simulink model "get_pluse_data"  (R2022a)
settings: Solver=FixedStepAuto  StartTime=0.0  StopTime=0.03  FixedStep=0.001  RelTol=1e-3
settings Model: Creator=12496  LastModifiedBy=12496

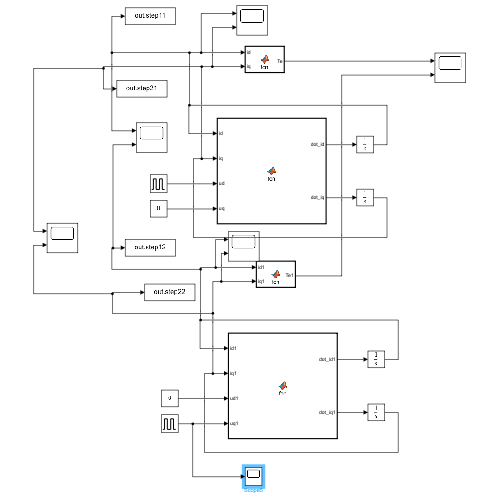
[thumbnail: Simulink's stored preview of the top-level diagram]
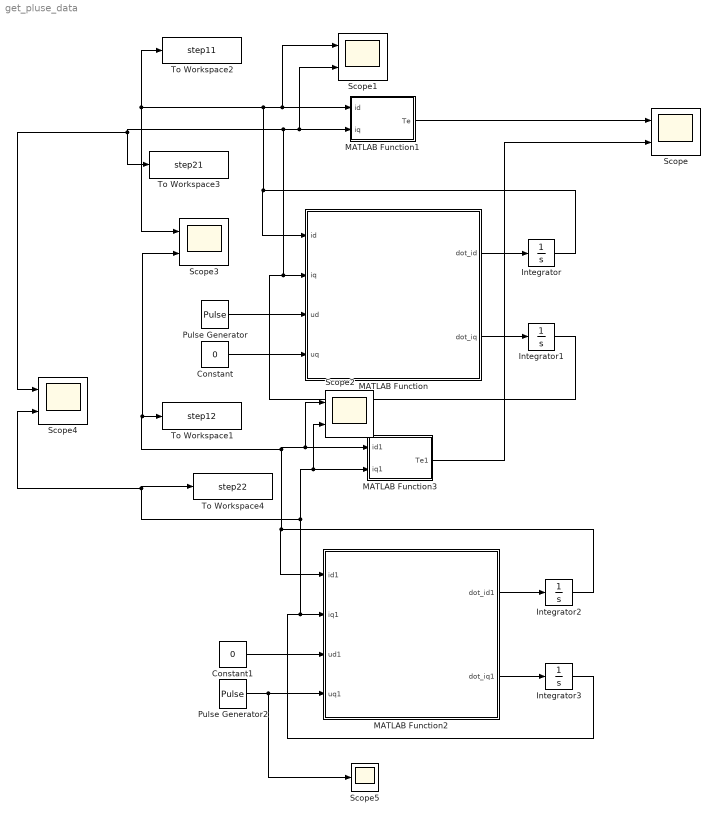
== system get_pluse_data ==
  Constant : Constant  Value=0
  Constant1 : Constant  Value=0
  Integrator{,1..3} (4 alike) : Integrator
  MATLAB Function : MATLAB Function  TreatAsAtomicUnit=on
  MATLAB Function1 : MATLAB Function  TreatAsAtomicUnit=on
  MATLAB Function2 : MATLAB Function  TreatAsAtomicUnit=on
  MATLAB Function3 : MATLAB Function  TreatAsAtomicUnit=on
  Pulse Generator : DiscretePulseGenerator  PulseType=Time based  Period=1  PulseWidth=0.1  PhaseDelay=0.005
  Pulse Generator2 : DiscretePulseGenerator  PulseType=Time based  Period=1  PulseWidth=0.1  PhaseDelay=0.005
  Scope{,1..4} (5 alike) : Scope  NumInputPorts=2
  Scope5 : Scope
  To Workspace1 : ToWorkspace  VariableName=step12  SampleTime=-1
  To Workspace2 : ToWorkspace  VariableName=step11  SampleTime=-1
  To Workspace3 : ToWorkspace  VariableName=step21  SampleTime=-1
  To Workspace4 : ToWorkspace  VariableName=step22  SampleTime=-1
  wires:
  MATLAB Function/1(dot_id) -> Integrator/1
  MATLAB Function/2(dot_iq) -> Integrator1/1
  Pulse Generator/1 -> MATLAB Function/3(ud)
  Constant/1 -> MATLAB Function/4(uq)
  Integrator/1 -> Scope3/1, To Workspace2/1, Scope1/1, MATLAB Function1/1(id), MATLAB Function/1(id)
  Integrator1/1 -> Scope4/1, To Workspace3/1, Scope1/2, MATLAB Function1/2(iq), MATLAB Function/2(iq)
  MATLAB Function1/1(Te) -> Scope/1
  MATLAB Function3/1(Te1) -> Scope/2
  MATLAB Function2/1(dot_id1) -> Integrator2/1
  Integrator2/1 -> MATLAB Function2/1(id1), Scope3/2, To Workspace1/1, Scope2/1, MATLAB Function3/1(id1)
  Integrator3/1 -> Scope4/2, To Workspace4/1, Scope2/2, MATLAB Function3/2(iq1), MATLAB Function2/2(iq1)
  MATLAB Function2/2(dot_iq1) -> Integrator3/1
  Constant1/1 -> MATLAB Function2/3(ud1)
  Pulse Generator2/1 -> Scope5/1, MATLAB Function2/4(uq1)

== matlab function get_pluse_data/MATLAB Function1 ==
  data: id input; Te output; iq input
function Te = fcn(id,iq)
Pn=4; %电机极对数
Fai=0.175; %转子磁链

C = [0 3*Pn*Fai/2];
Te=C*[id;iq];

== matlab function get_pluse_data/MATLAB Function ==
  data: id input; dot_id output; iq input; ud input; uq input; dot_iq output
function [dot_id,dot_iq] = fcn(id,iq,ud,uq)
Ld=0.0085;
Lq=0.0085;
R=2.875; %定子电阻
Pn=4; %电机极对数
Omega=100; %电机机械转速(单位:rad/s)
Fai=0.175; %转子磁链

A = [-R/Ld Pn*Omega*Lq/Ld;-Pn*Omega*Ld/Lq -R/Lq];
B = [1/Ld 0;0 1/Lq];
x=[id;iq];
u=[ud;uq];
dotx=A*x+B*u-[0;Pn*Omega*Fai/Lq];
dot_id=dotx(1);
dot_iq=dotx(2);

== matlab function get_pluse_data/MATLAB Function2 ==
  data: id1 input; dot_id1 output; iq1 input; ud1 input; uq1 input; dot_iq1 output
function [dot_id1,dot_iq1] = fcn(id1,iq1,ud1,uq1)
Ld=0.0085;
Lq=0.0085;
R=2.875; %定子电阻
Pn=4; %电机极对数
Omega=100; %电机机械转速(单位:rad/s)
Fai=0.175; %转子磁链

A = [-R/Ld Pn*Omega*Lq/Ld;-Pn*Omega*Ld/Lq -R/Lq];
B = [1/Ld 0;0 1/Lq];
x1=[id1;iq1];
u1=[ud1;uq1];
dotx1=A*x1+B*u1-[0;Pn*Omega*Fai/Lq];
dot_id1=dotx1(1);
dot_iq1=dotx1(2);

== matlab function get_pluse_data/MATLAB Function3 ==
  data: id1 input; Te1 output; iq1 input
function Te1 = fcn(id1,iq1)
Pn=4; %电机极对数
Fai=0.175; %转子磁链

C = [0 3*Pn*Fai/2];
Te1=C*[id1;iq1];
